simulink model "MODELO_MPC"  (R2025b)
settings: Solver=FixedStepDiscrete  StartTime=0.0  StopTime=8000  MaxStep=1.0  RelTol=1e-3
values from neighbouring files (symbols this model uses):
  Amd = A    [setup_MPC_NN_simple_v5.m]
  B_all = [Bm Bmd]    [setup_MPC_NN_simple_v5.m]
  Cmd = C    [setup_MPC_NN_simple_v5.m]
  D_all = zeros(size(C,1),1+4)    [setup_MPC_NN_simple_v5.m]
undefined symbols (not defined in the file or in its folder): dspblkCoreblockFVToolHelper, gcbh
libraries: mpclib x1
settings Model: PacingRate=100  Creator=Usuario  LastModifiedBy=Usuario

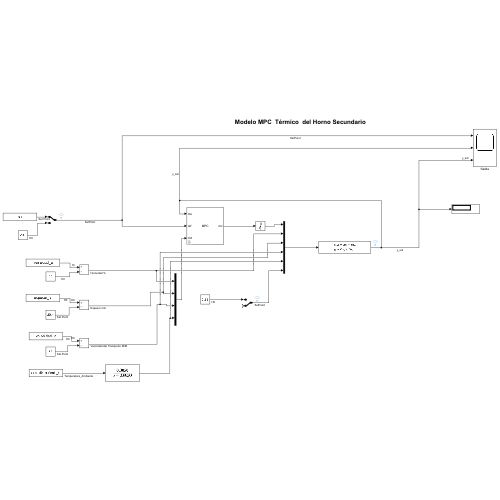
[thumbnail: Simulink's stored preview of the top-level diagram]
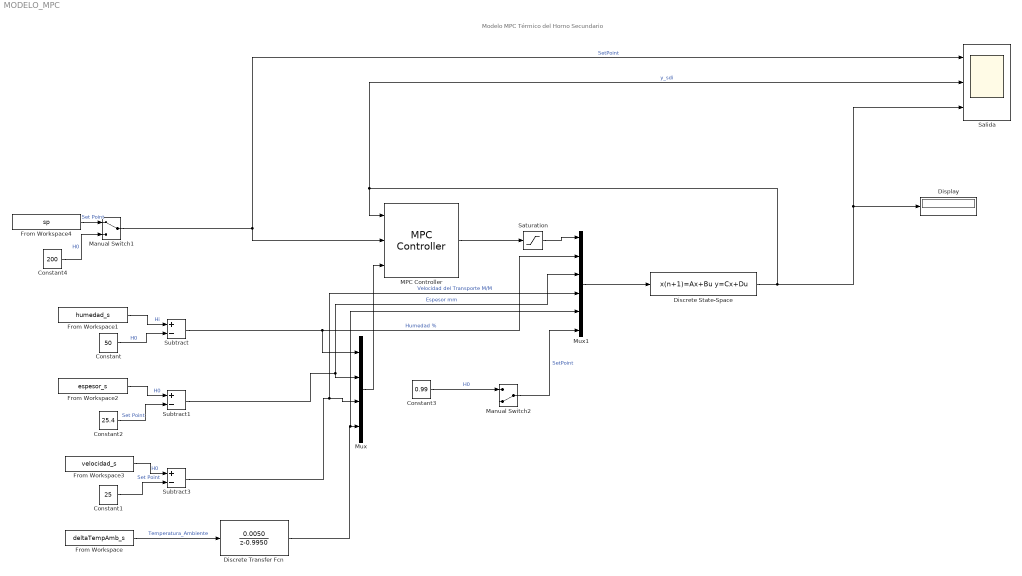
== system MODELO_MPC ==
  note: Modelo MPC Térmico del Horno Secundario
  Constant : Constant  Value=50
  Constant1 : Constant  Value=25
  Constant2 : Constant  Value=25.4
  Constant3 : Constant  Value=0.99
  Constant4 : Constant  Value=200
  Discrete Transfer Fcn : DiscreteTransferFcn  LoadFcn=dspblkCoreblockFVToolHelper(gcbh,'load');  Numerator=[0 0.0050]  Denominator=[1 -0.9950]
      settings: CopyFcn=dspblkCoreblockFVToolHelper(gcbh,'copy');  DeleteFcn=dspblkCoreblockFVToolHelper(gcbh,'close');  ModelCloseFcn=dspblkCoreblockFVToolHelper(gcbh,'close');  PreSaveFcn=dspblkCoreblockFVToolHelper(gcbh,'presave');  PostSaveFcn=dspblkCoreblockFVToolHelper(gcbh,'postsave');  CloseFcn=dspblkCoreblockFVToolHelper(gcbh,'close');
  Discrete State-Space : DiscreteStateSpace  A=Amd  B=B_all  C=Cmd  D=D_all
  Display : Display
      settings: Decimation=3
  From Workspace : FromWorkspace  VariableName=deltaTempAmb_s  OutputAfterFinalValue=Holding final value
  From Workspace1 : FromWorkspace  VariableName=humedad_s  OutputAfterFinalValue=Holding final value
  From Workspace2 : FromWorkspace  VariableName=espesor_s  OutputAfterFinalValue=Holding final value
  From Workspace3 : FromWorkspace  VariableName=velocidad_s  OutputAfterFinalValue=Holding final value
  From Workspace4 : FromWorkspace  VariableName=sp  OutputAfterFinalValue=Holding final value
  MPC Controller : mpclib/MPC Controller  SCDEnableBlockLinearizationSpecification=on  mpcobj=mpcobj  is_multiple=0  enable_value=0  return_u0=off  updateMPCinCallerWorkspace=on  md_inport=on  mv_inport=off  uref_inport=off  return_cost=off  return_mvseq=off  return_qpstatus=off  return_xseq=off  return_state=off  return_ovseq=off  state_inport=off  umin_inport=off  umax_inport=off  ymin_inport=off  ymax_inport=off  cc_inport=off  ywt_inport=off  uwt_inport=off  duwt_inport=off  rhoeps_inport=off  pm_inport=off  MaximumP=10  HorizonChoice=FixedHorizon  n_ts=1  n_p=18  n_mv=1  n_md=4  n_ud=1  n_mo=1  n_uo=0  BlockDataType=double  SampleTimeInherited=off  switch_inport=off
  Manual Switch1 : ManualSwitch
  Manual Switch2 : ManualSwitch  CurrentSetting=0
  Mux : Mux
  Mux1 : Mux  Inputs=6
  Salida : Scope  NumInputPorts=3
      settings: ActiveDisplayYMinimum=27.792171201159192  ActiveDisplayYMaximum=334.68575661195723  DataLoggingVariableName=ScopeData2
  Saturation : Saturate  UpperLimit=1.8  LowerLimit=0
  Subtract : Sum  Inputs=+-
  Subtract1 : Sum  Inputs=+-
  Subtract3 : Sum  Inputs=+-
  wires:
  Manual Switch1/1 -> MPC Controller/2, Salida/1  "SetPoint"
  From Workspace1/1 -> Subtract/1  "Hi"
  Discrete State-Space/1 -> MPC Controller/1, Salida/2, Salida/3, Display/1  "y_sdi"
  Constant2/1 -> Subtract1/2  "Set Point"
  Constant/1 -> Subtract/2  "H0"
  Constant1/1 -> Subtract3/2  "Set Point"
  Discrete Transfer Fcn/1 -> Mux1/5, Mux/4
  Subtract1/1 -> Mux1/3, Mux/2  "Espesor mm"
  From Workspace/1 -> Discrete Transfer Fcn/1  "Temperatura_Ambiente"
  Subtract3/1 -> Mux1/4, Mux/3  "Velocidad del Transporte M/M"
  From Workspace2/1 -> Subtract1/1  "H0"
  Subtract/1 -> Mux1/2, Mux/1  "Humedad %"
  From Workspace3/1 -> Subtract3/1  "H0"
  Mux/1 -> MPC Controller/3
  MPC Controller/1 -> Saturation/1
  Saturation/1 -> Mux1/1
  Mux1/1 -> Discrete State-Space/1
  From Workspace4/1 -> Manual Switch1/1  "Set Point"
  Constant4/1 -> Manual Switch1/2  "H0"
  Constant3/1 -> Manual Switch2/1  "H0"
  Manual Switch2/1 -> Mux1/6  "SetPoint"
